simulink model "Sender_Final"  (R2023b)
settings: Solver=FixedStepAuto  StartTime=0.0  StopTime=10.0  RelTol=1e-3
libraries: androidsensorlib x2, androidaudiovideolib x1, androidcommunicationlib x1, dspsigops x1
settings Model: Creator=hp  LastModifiedBy=krish
settings OptimizationCC: EnhancedBackFolding=on  PassReuseOutputArgsThreshold=0  MaxStackSize=64  OptimizeBlockOrder=speed  DifferentSizesBufferReuse=on  OptimizationCustomize=off
settings DebuggingCC: ParameterTunabilityLossMsg=error
settings HardwareCC: ProdBitPerLong=64  ProdLargestAtomicInteger=LongLong  ProdLargestAtomicFloat=Double  ProdLongLongMode=on  ProdHWDeviceType=ARM Compatible->ARM Cortex-A (64-bit)  UseEmbeddedCoderFeatures=off  UseSimulinkCoderFeatures=off
settings SFSimCC: MATLABDynamicMemAlloc=off
settings RTWCC: Description=Embedded Coder  SystemTargetFile=ert.tlc  HardwareBoard=Android Device (64bit)  TLCOptions="-aInlineSetEventsForThisBaseRateFcn=TLC_FALSE -aSuppressMultiTaskScheduler=TLC_FALSE  -aRateBasedStepFcn=0"  TemplateMakefile=ert_default_tmf  RTWVerbose=off  Toolchain=Android SDK/NDK Tools
settings CodeAppCC: ForceParamTrailComments=on  OperatorAnnotations=on
settings ERTTargetCC: ERTCustomFileBanners=off  SupportContinuousTime=on  SupportNonInlinedSFcns=on  RemoveResetFunc=off  ModelStepFunctionPrototypeControlCompliant=off

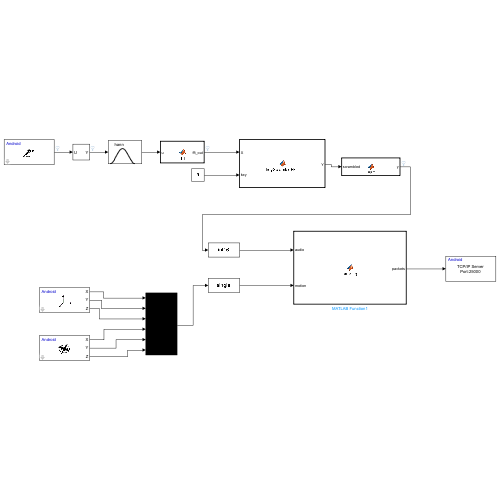
[thumbnail: Simulink's stored preview of the top-level diagram]
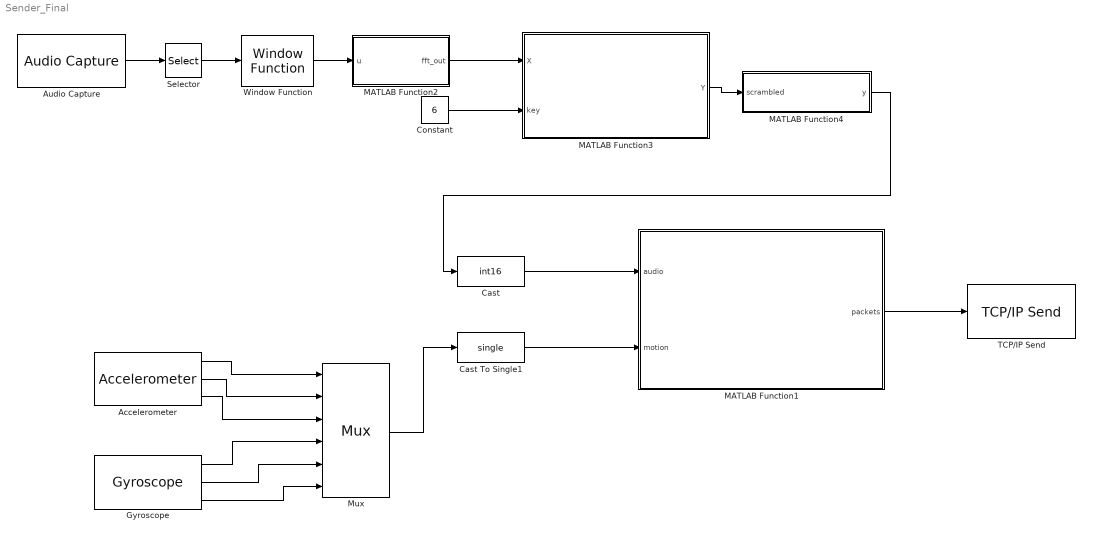
== system Sender_Final ==
  Accelerometer : androidsensorlib/Accelerometer  OutputVector=off  SampleTime=0.1  BlockPlatform=Android
  Audio Capture : androidaudiovideolib/Audio Capture  SampleFreq=44100  FrameSize=4410  SampleTime=0.1  SimulateUsing=Code generation  DeviceStr=0  QueueDuration=0  BlockPlatform=Android  AudioSamplingFreq=44100
  Cast : DataTypeConversion  OutDataTypeStr=int16  SaturateOnIntegerOverflow=off  RndMeth=Floor
  Cast To Single1 : DataTypeConversion  OutDataTypeStr=single  SaturateOnIntegerOverflow=off  RndMeth=Floor
  Constant : Constant  Value=6
  Gyroscope : androidsensorlib/Gyroscope  OutputVector=off  SampleTime=0.1  BlockPlatform=Android
  MATLAB Function1 : MATLAB Function  TreatAsAtomicUnit=on
  MATLAB Function2 : MATLAB Function  TreatAsAtomicUnit=on
  MATLAB Function3 : MATLAB Function  TreatAsAtomicUnit=on
  MATLAB Function4 : MATLAB Function  TreatAsAtomicUnit=on
  Mux : Mux  Inputs=6
  Selector : Selector  NumberOfDimensions=2  InputPortWidth=3  IndexOptions=Select all,Index vector (dialog)  Indices=[1 3],1  OutputSizes=1,1
  TCP/IP Send : androidcommunicationlib/TCP//IP Send  TCPSendId=Hasan_Sender/TCP//IP_Send  Mode_=Server  LocalServerPort_=25000  RemoteAddr_=127.0.0.1  RemoteServerPort_=25000  ClientPortBindingSelection_=off  ClientPortToBind_=35000  BlockingMode_=off  BlockTimeout_=0.1
  Window Function : dspsigops/Window Function  winmode=Apply window to input  wintype=Hann  sampmode=Continuous  samptime=1  N=64  Rs=50  beta=10  winsamp=Symmetric  UserWindow=hamming  OptParams=off  UserParams={'symmetric'}  dataType=double  isSigned=on  wordLen=16  udDataType=sfix(16)  fracBitsMode=Best precision  numFracBits=15  roundingMode=Floor  overflowMode=off  numSidelobes=4  sidelobeLevel=-30
  wires:
  Cast/1 -> MATLAB Function1/1(audio)
  Accelerometer/1 -> Mux/1
  Accelerometer/2 -> Mux/2
  Accelerometer/3 -> Mux/3
  Gyroscope/1 -> Mux/4
  Gyroscope/2 -> Mux/5
  Gyroscope/3 -> Mux/6
  Mux/1 -> Cast To Single1/1
  Cast To Single1/1 -> MATLAB Function1/2(motion)
  MATLAB Function1/1(packets) -> TCP/IP Send/1
  Selector/1 -> Window Function/1
  MATLAB Function4/1(y) -> Cast/1
  Audio Capture/1 -> Selector/1
  Window Function/1 -> MATLAB Function2/1(u)
  MATLAB Function2/1(fft_out) -> MATLAB Function3/1(X)
  MATLAB Function3/1(Y) -> MATLAB Function4/1(scrambled)
  Constant/1 -> MATLAB Function3/2(key)

== matlab function Sender_Final/MATLAB Function2 ==
  data: u input; fft_out output
function fft_out = FFT(u)
    u = u(:,1);
    fft_out = fft(double(u));
end

== matlab function Sender_Final/MATLAB Function3 ==
  data: X input; Y output; key input
function Y = keyScrambleFFT(X, key)
    [N, C] = size(X);

    posIdx = 2:floor(N/2);
    negIdx = N - posIdx + 2;

    K = numel(posIdx);
    if K == 0
        Y = X;
        return;
    end

    b = mod(key, K);
    a = mod(key, K-1) + 1;
    while K > 1 && gcd(a, K) ~= 1
        a = a + 1;
        if a >= K
            a = 1;
        end
    end

    perm = zeros(1, K);
    for i = 0:(K-1)
        perm(i+1) = mod(a * i + b, K) + 1;
    end

    pidx = posIdx(perm);    
    if ~isreal(X)
        Y = complex(zeros(N, C, 'like', X));
    else
        Y = zeros(N, C, 'like', X);
    end

    Y(1, :) = X(1, :);
    if mod(N,2) == 0
        Y(N/2 + 1, :) = X(N/2 + 1, :);
    end

    Y(posIdx, :) = X(pidx, :);

    if ~isreal(X)
        Y(negIdx, :) = conj(Y(posIdx, :));
    else
        Y(negIdx, :) = Y(posIdx, :);
    end
end

== matlab function Sender_Final/MATLAB Function4 ==
  data: scrambled input; y output
function y = IFFT(scrambled)
    N = length(scrambled);
    scrambled(2:N/2) = conj(scrambled(N:-1:N/2+2));
    Channel = ifft(scrambled);
    y = real(Channel);
end

== matlab function Sender_Final/MATLAB Function1 ==
  data: audio input; packets output; motion input
function packets = packing(audio, motion)
assert(isa(motion,'single') && numel(motion)==6);
assert(isa(audio,'int16') && numel(audio)==4410);

packets = zeros(8844,1,'uint8');   % total = 24 + 8820

packets(1:24)    = typecast(motion(:), 'uint8').';        
packets(25:8844) = typecast(audio(:), 'uint8').';
end
